simulink model "matlab_pid_dealy_smith_9"  (R2018b)
settings: Solver=VariableStepAuto  StartTime=0.0  StopTime=40  RelTol=1e-3
libraries: simulink x2
settings Model: Creator=erange  LastModifiedBy=erange

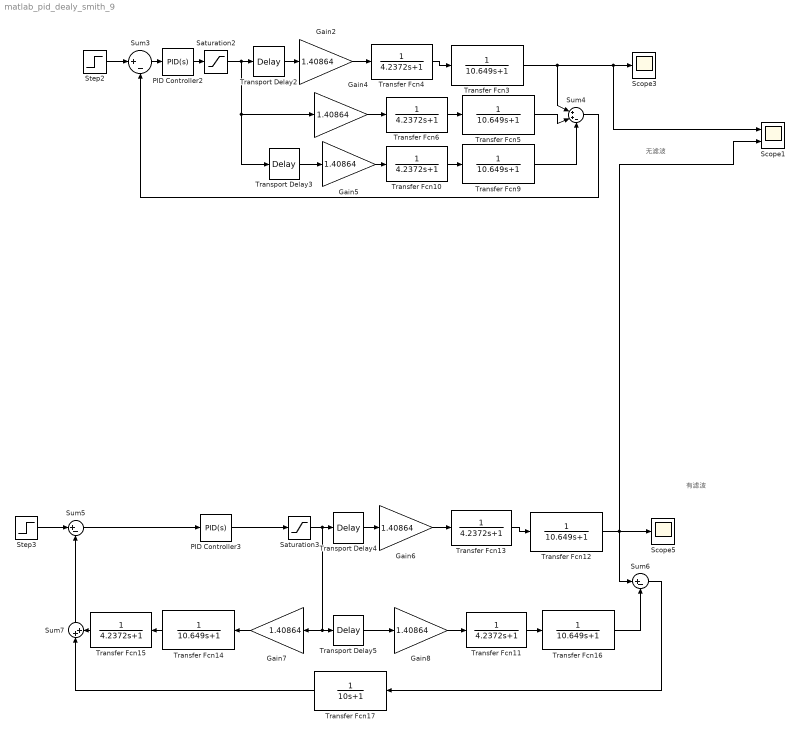
== system matlab_pid_dealy_smith_9 ==
  note: 有滤波
  note: 无滤波
  Gain{2,4..8} (6 alike) : Gain  Gain=1.40864
  PID Controller2 : simulink/Continuous/PID Controller  Controller=PID  Form=Ideal  TimeDomain=Continuous-time  SampleTime=0.1  IntegratorMethod=Forward Euler  FilterMethod=Forward Euler  ControllerParametersSource=internal  P=5  I=0.1  D=1.5  UseFilter=on  N=10000  TunerSelectOption=Transfer Function Based (PID Tuner App)  InitialConditionSource=internal  InitialConditionForIntegrator=0  InitialConditionForFilter=0  DifferentiatorICPrevScaledInput=0  ExternalReset=none  TrackingMode=off  Kt=1  LimitOutput=off  UpperSaturationLimit=inf  LowerSaturationLimit=-inf  LinearizeAsGain=on  AntiWindupMode=none  Kb=1  POutMin=[]  POutMax=[]  IOutMin=[]  IOutMax=[]  DOutMin=[]  DOutMax=[]  NOutMin=[]  NOutMax=[]  SumOutMin=[]  SumOutMax=[]  SaturationOutMin=[]  SaturationOutMax=[]  PParamMin=[]  PParamMax=[]  IParamMin=[]  IParamMax=[]  DParamMin=[]  DParamMax=[]  NParamMin=[]  NParamMax=[]  KbParamMin=[]  KbParamMax=[]  KtParamMin=[]  KtParamMax=[]  KbOutMin=[]  KbOutMax=[]  KtOutMin=[]  KtOutMax=[]  IntegratorOutMin=[]  IntegratorOutMax=[]  FilterOutMin=[]  FilterOutMax=[]  SumI1OutMin=[]  SumI1OutMax=[]  SumI2OutMin=[]  SumI2OutMax=[]  SumI3OutMin=[]  SumI3OutMax=[]  SumI4OutMin=[]  SumI4OutMax=[]  SumDOutMin=[]  SumDOutMax=[]  DifferentiatorOutMin=[]  DifferentiatorOutMax=[]  FilterDiffOutCoefMin=[]  FilterDiffOutCoefMax=[]  ReciprocalOutMin=[]  ReciprocalOutMax=[]  SumDenOutMin=[]  SumDenOutMax=[]  SumNumOutMin=[]  SumNumOutMax=[]  DivideOutMin=[]  DivideOutMax=[]  IntegratorContinuousStateAttributes=''  IntegratorStateMustResolveToSignalObject=off  IntegratorRTWStateStorageClass=Auto  FilterContinuousStateAttributes=''  FilterStateMustResolveToSignalObject=off  FilterRTWStateStorageClass=Auto  ParallelPVariant=Passthrough  IdealPVariant=InternalParameters  IVariant=InternalParameters  DVariant=InternalParameters  IntegratorVariant=Continuous  SatVariant=Disabled  AWVariant=Passthrough  PCopyVariant=Disabled  TRVariant=Disabled  FdbkBlocksVariant=Forward  IdealPFdbkVariant=Disabled  SatFdbkVariant=Disabled  DerivativeFilterVariant=ContFilter  NVariant=InternalParameters  NCopyVariant=Disabled  FilterICVariant=InternalICsFilter  IntegratorICVariant=InternalICs  ExternalResetVariant=Disabled  TRSumVariant=Passthrough  SumFdbkVariant=Disabled  SumVariant=Sum_PID
  PID Controller3 : simulink/Continuous/PID Controller  Controller=PID  Form=Ideal  TimeDomain=Continuous-time  SampleTime=0.1  IntegratorMethod=Forward Euler  FilterMethod=Forward Euler  ControllerParametersSource=internal  P=5  I=0.1  D=1.5  UseFilter=on  N=10000  TunerSelectOption=Transfer Function Based (PID Tuner App)  InitialConditionSource=internal  InitialConditionForIntegrator=0  InitialConditionForFilter=0  DifferentiatorICPrevScaledInput=0  ExternalReset=none  TrackingMode=off  Kt=1  LimitOutput=off  UpperSaturationLimit=inf  LowerSaturationLimit=-inf  LinearizeAsGain=on  AntiWindupMode=none  Kb=1  POutMin=[]  POutMax=[]  IOutMin=[]  IOutMax=[]  DOutMin=[]  DOutMax=[]  NOutMin=[]  NOutMax=[]  SumOutMin=[]  SumOutMax=[]  SaturationOutMin=[]  SaturationOutMax=[]  PParamMin=[]  PParamMax=[]  IParamMin=[]  IParamMax=[]  DParamMin=[]  DParamMax=[]  NParamMin=[]  NParamMax=[]  KbParamMin=[]  KbParamMax=[]  KtParamMin=[]  KtParamMax=[]  KbOutMin=[]  KbOutMax=[]  KtOutMin=[]  KtOutMax=[]  IntegratorOutMin=[]  IntegratorOutMax=[]  FilterOutMin=[]  FilterOutMax=[]  SumI1OutMin=[]  SumI1OutMax=[]  SumI2OutMin=[]  SumI2OutMax=[]  SumI3OutMin=[]  SumI3OutMax=[]  SumI4OutMin=[]  SumI4OutMax=[]  SumDOutMin=[]  SumDOutMax=[]  DifferentiatorOutMin=[]  DifferentiatorOutMax=[]  FilterDiffOutCoefMin=[]  FilterDiffOutCoefMax=[]  ReciprocalOutMin=[]  ReciprocalOutMax=[]  SumDenOutMin=[]  SumDenOutMax=[]  SumNumOutMin=[]  SumNumOutMax=[]  DivideOutMin=[]  DivideOutMax=[]  IntegratorContinuousStateAttributes=''  IntegratorStateMustResolveToSignalObject=off  IntegratorRTWStateStorageClass=Auto  FilterContinuousStateAttributes=''  FilterStateMustResolveToSignalObject=off  FilterRTWStateStorageClass=Auto  ParallelPVariant=Passthrough  IdealPVariant=InternalParameters  IVariant=InternalParameters  DVariant=InternalParameters  IntegratorVariant=Continuous  SatVariant=Disabled  AWVariant=Passthrough  PCopyVariant=Disabled  TRVariant=Disabled  FdbkBlocksVariant=Forward  IdealPFdbkVariant=Disabled  SatFdbkVariant=Disabled  DerivativeFilterVariant=ContFilter  NVariant=InternalParameters  NCopyVariant=Disabled  FilterICVariant=InternalICsFilter  IntegratorICVariant=InternalICs  ExternalResetVariant=Disabled  TRSumVariant=Passthrough  SumFdbkVariant=Disabled  SumVariant=Sum_PID
  Saturation2 : Saturate  UpperLimit=5  LowerLimit=0
  Saturation3 : Saturate  UpperLimit=5  LowerLimit=0
  Scope1 : Scope  NumInputPorts=2
  Scope3 : Scope
  Scope5 : Scope
  Step2 : Step  Time=0  SampleTime=1
  Step3 : Step  Time=0  SampleTime=1
  Sum3 : Sum  Inputs=|+-
  Sum4 : Sum  Inputs=|++-
  Sum5 : Sum  Inputs=|+-
  Sum6 : Sum  Inputs=|+-
  Sum7 : Sum  Inputs=|++
  Transfer Fcn{4,6,10..11,13,15} (6 alike) : TransferFcn  Denominator=[4.2372 1]
  Transfer Fcn{3,5,9,12,14,16} (6 alike) : TransferFcn  Denominator=[10.649 1]
  Transfer Fcn17 : TransferFcn  Denominator=[10 1]
  Transport Delay{2..5} (4 alike) : TransportDelay  DelayTime=3
  wires:
  Transport Delay2/1 -> Gain2/1
  Step2/1 -> Sum3/1
  Gain2/1 -> Transfer Fcn4/1
  Transfer Fcn4/1 -> Transfer Fcn3/1
  Sum3/1 -> PID Controller2/1
  Transfer Fcn6/1 -> Transfer Fcn5/1
  Gain4/1 -> Transfer Fcn6/1
  Gain5/1 -> Transfer Fcn10/1
  Transfer Fcn10/1 -> Transfer Fcn9/1
  Transport Delay3/1 -> Gain5/1
  Sum4/1 -> Sum3/2
  Transfer Fcn5/1 -> Sum4/2
  Transfer Fcn13/1 -> Transfer Fcn12/1
  Transfer Fcn12/1 -> Scope5/1, Scope1/2, Sum6/1
  Gain6/1 -> Transfer Fcn13/1
  Gain8/1 -> Transfer Fcn11/1
  PID Controller3/1 -> Saturation3/1
  Transport Delay5/1 -> Gain8/1
  Transport Delay4/1 -> Gain6/1
  Step3/1 -> Sum5/1
  Sum5/1 -> PID Controller3/1
  Saturation3/1 -> Gain7/1, Transport Delay5/1, Transport Delay4/1
  Transfer Fcn11/1 -> Transfer Fcn16/1
  Transfer Fcn16/1 -> Sum6/2
  Transfer Fcn14/1 -> Transfer Fcn15/1
  Gain7/1 -> Transfer Fcn14/1
  Transfer Fcn15/1 -> Sum7/2
  Sum7/1 -> Sum5/2
  Sum6/1 -> Transfer Fcn17/1
  Transfer Fcn17/1 -> Sum7/1
  Transfer Fcn3/1 -> Scope3/1, Scope1/1, Sum4/1
  Transfer Fcn9/1 -> Sum4/3
  PID Controller2/1 -> Saturation2/1
  Saturation2/1 -> Transport Delay3/1, Gain4/1, Transport Delay2/1
